simulink model "AccTarSel"  (R2018b)
settings: Solver=FixedStepDiscrete  StartTime=0.0  StopTime=inf  FixedStep=0.01  RelTol=1e-3
PostLoadFcn:
  | if any(exist('dsrtsu_mdlpostloadfcn', 'file') ~= 0), dsrtsu_mdlpostloadfcn('Execute', bdroot); end
values from neighbouring files (symbols this model uses):
  P_adtMaxBDC = 1.0    [AccTarSel.sldd]
  P_aFOCApproachIntpAcitve = -0.6    [AccTarSel.sldd]
  P_aFOCApproachIntpEnsure = -1.8    [AccTarSel.sldd]
  P_CutInEnable = 1.0    [AccTarSel.sldd]
  P_dAimMin = 4.5    [AccTarSel.sldd]
  P_dAimMinAVP = 1.5    [AccTarSel.sldd]
  P_dObjDrvOffMax = 5.0    [AccTarSel.sldd]
  P_dObjDrvOffMin = 3.0    [AccTarSel.sldd]
  P_dObjLowHystDecToStop = 4.5    [AccTarSel.sldd]
  P_dObjLowHystDecToStopAVP = 1.5    [AccTarSel.sldd]
  P_dObjUpperHystDecToStop = 5.0    [AccTarSel.sldd]
  P_dResMax = 5.0    [AccTarSel.sldd]
  P_dStandStill = 3.0    [AccTarSel.sldd]
  P_dStandStillMin = 2.0    [AccTarSel.sldd]
  P_dvarYMax4PO = 1.0    [AccTarSel.sldd]
  P_dyCutInThres = 3.6    [AccTarSel.sldd]
  P_facBDCInit = 0.7    [AccTarSel.sldd]
  P_facBDCIterCalc = 0.8    [AccTarSel.sldd]
  P_facFOCNegDiff = 0.3    [AccTarSel.sldd]
  P_facFOCPosDiff = 0.2    [AccTarSel.sldd]
  P_kapHystThres = 0.0005    [AccTarSel.sldd]
  P_PlausIntegDisable = 0.0    [AccTarSel.sldd]
  P_plausMin4PO = 0.5    [AccTarSel.sldd]
  P_probExistMin4PO = 0.8    [AccTarSel.sldd]
  P_StandObjEnable = 0.0    [AccTarSel.sldd]
  P_tAxTrackNegLower = 0.3    [AccTarSel.sldd]
  P_tAxTrackNegUpper = 0.6    [AccTarSel.sldd]
  P_tAxTrackPosLower = 1.0    [AccTarSel.sldd]
  P_tAxTrackPosUpper = 2.0    [AccTarSel.sldd]
  P_tBDCStartFilt = 0.2    [AccTarSel.sldd]
  P_tCSC = 3.5    [AccTarSel.sldd]
  P_tCurvFilt = 0.2    [AccTarSel.sldd]
  P_tCutInFilt = 0.5    [AccTarSel.sldd]
  P_tFiltAxAbsPONegFast = 0.1    [AccTarSel.sldd]
  P_tFiltAxAbsPONegSlow = 0.4    [AccTarSel.sldd]
  P_tFiltAxAbsPOPosFast = 1.2    [AccTarSel.sldd]
  P_tFiltAxAbsPOPosSlow = 2.0    [AccTarSel.sldd]
  P_tFiltAxAbsPOStand = 2.0    [AccTarSel.sldd]
  P_tFiltDAim = 0.1    [AccTarSel.sldd]
  P_tFiltDsd = 0.1    [AccTarSel.sldd]
  P_tFiltSpdLim = 3.0    [AccTarSel.sldd]
  P_tFiltVxAxPOFast = 0.15    [AccTarSel.sldd]
  P_tFiltVxAxPOSlow = 0.25    [AccTarSel.sldd]
  P_tFOCStatAccelFast = 4.0    [AccTarSel.sldd]
  P_tFOCStatAccelSlow = 3.5    [AccTarSel.sldd]
  P_tFOCStatDecelFast = 4.0    [AccTarSel.sldd]
  P_tFOCStatDecelSlow = 3.2    [AccTarSel.sldd]
  P_tMinDrvPhase = 2.0    [AccTarSel.sldd]
  P_tPredObjLeav = 1.2    [AccTarSel.sldd]
  P_tRollingFilt = 0.5    [AccTarSel.sldd]
  P_tRollingFinFilt = 1.0    [AccTarSel.sldd]
  P_tSSCNeg = 4.5    [AccTarSel.sldd]
  P_tSSCPos = 5.5    [AccTarSel.sldd]
  P_tToStop = 5.0    [AccTarSel.sldd]
  P_tToStopInBDC = 6.0    [AccTarSel.sldd]
  P_tToStopTrig = 4.0    [AccTarSel.sldd]
  P_vEgoDecToStop = 3.0    [AccTarSel.sldd]
  P_vEgoLowBDC = 4.0    [AccTarSel.sldd]
  P_vFOCNegDiff = 4.0    [AccTarSel.sldd]
  P_vFOCPosDiff = 5.0    [AccTarSel.sldd]
  P_vFOCStationaryFast = 15.0    [AccTarSel.sldd]
  P_vFOCStationarySlow = 5.0    [AccTarSel.sldd]
  P_vObjDrvOff = 0.5    [AccTarSel.sldd]
  P_vObjLowHystDecToStop = 0.5    [AccTarSel.sldd]
  P_vObjNoStop = 1.0    [AccTarSel.sldd]
  P_vObjReCalc = 1.0    [AccTarSel.sldd]
  P_vObjStop = 0.3    [AccTarSel.sldd]
  P_vObjUpperHystDecToStop = 0.8    [AccTarSel.sldd]
  P_vStandStill = 0.3    [AccTarSel.sldd]
  P_vStandStillHyst = 0.3    [AccTarSel.sldd]
  P_vyCutInThres = 0.5    [AccTarSel.sldd]
libraries: simulink x21, LPFilter x12
(part 10 of 11)

== system AccTarSel/ACC_Control/FollowObjCtrl/FollowObjValid/BrakeDistCtrl/calcCriteria/calcProfileReCalc ==
  note: should consider situation becomes urgent secnario later
  dObjToStop : Inport
  <vRef> : Inport  Port=2
  <aRef> : Inport  Port=3
  <dx> : Inport  Port=4
  vAbsObj : Inport  Port=5
  tElaps : Inport  Port=6
  BDC_StateK1 : Inport  Port=7
  ProfileK1 : Inport  Port=8
  AND : Logic  Inputs=3  AllPortsSameDT=off  OutDataTypeStr=boolean
  Abs : Abs
  Add2 : Sum  Inputs=++--
  Bus Creator : BusCreator  Inputs=5
  Bus Selector : BusSelector  OutputSignals=T30
  Constant : Constant  Value=-0.5  OutDataTypeStr=single
  Constant1 : Constant  Value=2  OutDataTypeStr=single
  Constant7 : Constant  Value=-0.3  OutDataTypeStr=single
  Constant8 : Constant  Value=2  OutDataTypeStr=single
  Divide2 : Product  Inputs=*/
  Min : MinMax  Inputs=2
  Multiply : Product
  OR : Logic  Operator=OR  Inputs=3  AllPortsSameDT=off  OutDataTypeStr=boolean
  P_dResMax : Constant  Value=P_dResMax  OutDataTypeStr=single
  P_dStandStill : Constant  Value=P_dStandStill  OutDataTypeStr=single
  P_vObjReCalc : Constant  Value=P_vObjReCalc  OutDataTypeStr=single
  Relational Operator : RelationalOperator  Operator===  OutDataTypeStr=boolean  RndMeth=Simplest
  Relational Operator1 : RelationalOperator  OutDataTypeStr=boolean  RndMeth=Simplest
  Relational Operator2 : RelationalOperator  Operator=<  OutDataTypeStr=boolean  RndMeth=Simplest
  Relational Operator4 : RelationalOperator  Operator=>  OutDataTypeStr=boolean  RndMeth=Simplest
  Relational Operator5 : RelationalOperator  Operator=>  OutDataTypeStr=boolean  RndMeth=Simplest
  Square : Math  Operator=square  SaturateOnIntegerOverflow=on
  To Workspace : ToWorkspace  VariableName=simout2  SaveFormat=Timeseries  SampleTime=-1
  ProfileReCalc : Outport
  dRes : Outport  Port=2
  wires:
  vAbsObj/1 -> Relational Operator5/1
  P_vObjReCalc/1 -> Relational Operator5/2
  P_dResMax/1 -> Relational Operator4/2
  Relational Operator5/1 -> OR/2
  P_dStandStill/1 -> Add2/4
  Add2/1 -> Relational Operator2/1, dRes/1, Bus Creator/5, Relational Operator4/1  "dRes"
  dObjToStop/1 -> Bus Creator/1, Add2/1
  Constant8/1 -> Multiply/2
  Min/1 -> Multiply/1
  <vRef>/1 -> Square/1
  Constant7/1 -> Min/2
  AND/1 -> ProfileReCalc/1
  Relational Operator4/1 -> OR/1
  Multiply/1 -> Divide2/2
  Square/1 -> Divide2/1
  <aRef>/1 -> Min/1
  <dx>/1 -> Bus Creator/2, Add2/2
  Divide2/1 -> Abs/1  "dEgoToStop"
  Abs/1 -> Add2/3
  Bus Creator/1 -> To Workspace/1
  BDC_StateK1/1 -> Relational Operator/1
  Constant1/1 -> Relational Operator/2
  ProfileK1/1 -> Bus Selector/1
  tElaps/1 -> Relational Operator1/1
  Bus Selector/1 -> Relational Operator1/2  "<T30>"
  OR/1 -> AND/1
  Relational Operator/1 -> AND/2
  Relational Operator1/1 -> AND/3, Bus Creator/4
  Constant/1 -> Relational Operator2/2
  Relational Operator2/1 -> OR/3

== system AccTarSel/ACC_Control/FollowObjCtrl/FollowObjValid/BrakeDistCtrl/calcProfile/If Action Subsystem ==
  In1 : Inport
  Action Port : ActionPort  ActionType=elseif
  Out1 : Outport
  wires:
  In1/1 -> Out1/1

== system AccTarSel/ACC_Control/FollowObjCtrl/FollowObjValid/BrakeDistCtrl/calcProfile/calc ==
  egoInfo : Inport
  objInfo : Inport  Port=2
  dObjToStop : Inport  Port=3
  aCvK1 : Inport  Port=4
  Action Port : ActionPort  ActionType=then
  Bus Creator : BusCreator  Inputs=7
  Relational Operator : RelationalOperator  OutDataTypeStr=boolean  RndMeth=Simplest
  Subsystem : Subsystem
  Switch : Switch  Criteria=u2 > Threshold
  calcInitCondition : Subsystem
  Profile : Outport
  wires:
  egoInfo/1 -> calcInitCondition/1(egoInfo)
  objInfo/1 -> calcInitCondition/2(objInfo)
  dObjToStop/1 -> calcInitCondition/3(dObjToStop)
  calcInitCondition/1(a0) -> Bus Creator/1, Switch/1, Relational Operator/1  "a0Raw"
  calcInitCondition/2(aThres) -> Switch/3, Relational Operator/2
  Relational Operator/1 -> Bus Creator/2, Switch/2  "SmoothStopCond"
  Switch/1 -> Bus Creator/3  "a0"
  calcInitCondition/3(v0) -> Bus Creator/4  "v0"
  calcInitCondition/4(v30) -> Bus Creator/5  "v30"
  calcInitCondition/5(dAimBDC) -> Bus Creator/6  "dAimBDC"
  calcInitCondition/6(d30) -> Bus Creator/7  "d30"
  Bus Creator/1 -> Subsystem/1(initCond)  "initCond"
  Subsystem/1(Profile) -> Profile/1
  aCvK1/1 -> calcInitCondition/4(aCvK1)

== system AccTarSel/ACC_Control/FollowObjCtrl/FollowObjValid/BrakeDistCtrl/calcProfile/default ==
  Action Port : ActionPort  ActionType=else
  Bus Creator : BusCreator  Inputs=8
  Constant{,1,3..7} (7 alike) : Constant  Value=0  OutDataTypeStr=single
  Constant2 : Constant  Value=0  OutDataTypeStr=boolean
  default : Outport
  wires:
  Bus Creator/1 -> default/1
  Constant1/1 -> Bus Creator/2  "aMax"
  Constant2/1 -> Bus Creator/1  "SmoothStopCond"
  Constant/1 -> Bus Creator/3  "T"
  Constant3/1 -> Bus Creator/4  "T30"
  Constant4/1 -> Bus Creator/5  "adt1"
  Constant5/1 -> Bus Creator/6  "adt2"
  Constant6/1 -> Bus Creator/7  "a0"
  Constant7/1 -> Bus Creator/8  "a0Raw"

== system AccTarSel/ACC_Control/FollowObjCtrl/FollowObjValid/FOC_MIX/Subsystem/If Action Subsystem ==
  aStat : Inport
  aApprh : Inport  Port=2
  Action Port : ActionPort  ActionType=then
  Min : MinMax  Inputs=2
  Out1 : Outport
  wires:
  aStat/1 -> Min/1
  aApprh/1 -> Min/2
  Min/1 -> Out1/1

== system AccTarSel/ACC_Control/FollowObjCtrl/FollowObjValid/FOC_MIX/Subsystem/If Action Subsystem1 ==
  aStat : Inport
  Action Port : ActionPort  ActionType=elseif
  Out1 : Outport
  wires:
  aStat/1 -> Out1/1

== system AccTarSel/ACC_Control/FollowObjCtrl/FollowObjValid/FOC_MIX/Subsystem/If Action Subsystem2 ==
  aStat : Inport
  aApprh : Inport  Port=2
  aActive : Inport  Port=3
  aEnsure : Inport  Port=4
  Action Port : ActionPort  ActionType=else
  Bus Creator : BusCreator  Inputs=2
  Bus Creator1 : BusCreator  Inputs=2
  Lookup Table Dynamic : simulink/Lookup Tables/Lookup Table Dynamic  LookUpMeth=Interpolation-Use End Values  OutDataType=fixdt('single')  OutScaling=[]  OutputDataTypeScalingMode=Specify via dialog  OutDataTypeStr=single  DoSatur=off
      settings: SourceProductName=Simulink
  Out1 : Outport
  wires:
  Bus Creator/1 -> Lookup Table Dynamic/2
  aApprh/1 -> Bus Creator1/1, Lookup Table Dynamic/1
  Bus Creator1/1 -> Lookup Table Dynamic/3
  Lookup Table Dynamic/1 -> Out1/1
  aEnsure/1 -> Bus Creator/1
  aActive/1 -> Bus Creator/2
  aStat/1 -> Bus Creator1/2

== system AccTarSel/ACC_Control/FollowObjCtrl/FollowObjValid/StationaryCtrl/calcCharactVal/If Action Subsystem ==
  dActual : Inport
  dBPNeg : Inport  Port=2
  Action Port : ActionPort  ActionType=then
  Abs : Abs
  Add : Sum  Inputs=+-
  Add1 : Sum
  Constant2 : Constant  Value=2  OutDataTypeStr=single
  Multiply : Product
  Multiply1 : Product
  Multiply2 : Product
  P_facFOCNegDiff : Constant  Value=P_facFOCNegDiff
  P_vFOCNegDiff : Constant  Value=P_vFOCNegDiff
  Sqrt : Sqrt  SaturateOnIntegerOverflow=on
  Square : Math  Operator=square  SaturateOnIntegerOverflow=on
  vUpper : Outport
  vLower : Outport  Port=2
  wires:
  dActual/1 -> Add/2
  P_facFOCNegDiff/1 -> Multiply/2
  dBPNeg/1 -> Add/1
  Sqrt/1 -> vUpper/1  "vUpper"
  Add/1 -> Multiply1/2
  Constant2/1 -> Multiply2/2
  Square/1 -> Add1/1
  Multiply2/1 -> Add1/2
  Abs/1 -> Multiply2/1
  P_vFOCNegDiff/1 -> vLower/1, Square/1, Multiply/1
  Multiply1/1 -> Abs/1
  Add1/1 -> Sqrt/1
  Multiply/1 -> Multiply1/1  "aConstNegPhase"

== system AccTarSel/ACC_Control/FollowObjCtrl/FollowObjValid/StationaryCtrl/calcCharactVal/If Action Subsystem4 ==
  dActual : Inport
  dAim : Inport  Port=2
  Action Port : ActionPort  ActionType=elseif
  Add : Sum  Inputs=+-
  Multiply : Product
  P_facFOCNegDiff : Constant  Value=P_facFOCNegDiff
  vUpper : Outport
  vLower : Outport  Port=2
  wires:
  dAim/1 -> Add/1
  dActual/1 -> Add/2
  P_facFOCNegDiff/1 -> Multiply/1
  Add/1 -> Multiply/2
  Multiply/1 -> vLower/1, vUpper/1

== system AccTarSel/ACC_Control/FollowObjCtrl/FollowObjValid/StationaryCtrl/calcCharactVal/If Action Subsystem5 ==
  dActual : Inport
  dAim : Inport  Port=2
  Action Port : ActionPort  ActionType=elseif
  Add : Sum  Inputs=+-
  Multiply : Product
  P_facFOCPosDiff : Constant  Value=P_facFOCPosDiff
  vUpper : Outport
  vLower : Outport  Port=2
  wires:
  Multiply/1 -> vUpper/1, vLower/1
  Add/1 -> Multiply/2
  P_facFOCPosDiff/1 -> Multiply/1
  dActual/1 -> Add/2
  dAim/1 -> Add/1

== system AccTarSel/ACC_Control/FollowObjCtrl/FollowObjValid/StationaryCtrl/calcCharactVal/If Action Subsystem6 ==
  dActual : Inport
  dBPPos : Inport  Port=2
  Action Port : ActionPort  ActionType=else
  Abs : Abs
  Add : Sum  Inputs=+-
  Add1 : Sum
  Constant : Constant  Value=-1  OutDataTypeStr=single
  Constant2 : Constant  Value=2  OutDataTypeStr=single
  Multiply{,1..4} (5 alike) : Product
  P_facFOCPosDiff : Constant  Value=P_facFOCPosDiff
  P_vFOCPosDiff : Constant  Value=P_vFOCPosDiff
  Sqrt : Sqrt  SaturateOnIntegerOverflow=on
  Square : Math  Operator=square  SaturateOnIntegerOverflow=on
  vUpper : Outport
  vLower : Outport  Port=2
  wires:
  Multiply/1 -> Multiply1/1  "aConstNegPhase"
  Add1/1 -> Sqrt/1
  Multiply1/1 -> Abs/1
  P_vFOCPosDiff/1 -> Multiply/1, Multiply3/1, Square/1
  Abs/1 -> Multiply2/1
  Multiply2/1 -> Add1/2
  Square/1 -> Add1/1
  Constant2/1 -> Multiply2/2
  Add/1 -> Multiply1/2
  P_facFOCPosDiff/1 -> Multiply/2
  dActual/1 -> Add/1
  dBPPos/1 -> Add/2
  Constant/1 -> Multiply3/2, Multiply4/1
  Sqrt/1 -> Multiply4/2  "vUpper"
  Multiply3/1 -> vUpper/1
  Multiply4/1 -> vLower/1

== system AccTarSel/ACC_Target_Selection/Subsystem/ValidObjCalc/CutInCalc/Subsystem/If Action Subsystem ==
  In1 : Inport
  Action Port : ActionPort  ActionType=else
  Constant : Constant  Value=0  OutDataTypeStr=single
  probCutInFiltInit : Outport
  dyCutInPredInit : Outport  Port=2
  probCutInRawInit : Outport  Port=3
  wires:
  Constant/1 -> probCutInRawInit/1, probCutInFiltInit/1
  In1/1 -> dyCutInPredInit/1

== system AccTarSel/ACC_Target_Selection/Subsystem/ValidObjCalc/CutInCalc/Subsystem/Subsystem ==
  note: MotionSts:
      | 0	Unknown
      | 1	Standstill
      | 2	Driving
      | 3	InvDriving
      | 4	Stopped
      | 5	InvStopped
  probCutInK1 : Inport
  dyToTraj : Inport  Port=2
  <vy> : Inport  Port=3
  MotionSts : Inport  Port=4
  SYS_Info_st : Inport  Port=5
  Action Port : ActionPort  ActionType=then
  Abs : Abs
  Abs1 : Abs
  Bus Selector : BusSelector  OutputSignals=dT
  Constant1 : Constant  Value=2  OutDataTypeStr=single
  Constant2 : Constant  Value=0
  If : If  IfExpression=u1 == 1
  If Action Subsystem : Subsystem  TreatAsAtomicUnit=on
  If Action Subsystem1 : Subsystem  TreatAsAtomicUnit=on
  LPFilter : LPFilter/LPFilter  SystemSampleTime=-1
      settings: SourceProductName=CustomLib
  Logical Operator : Logic  Inputs=5  AllPortsSameDT=off  OutDataTypeStr=boolean
  Merge : Merge
  Merge1 : Merge
  Multiply : Product
  P_CutInEnable : Constant  Value=P_CutInEnable
  P_dyCutInThres : Constant  Value=P_dyCutInThres
  P_tCutInFilt : Constant  Value=P_tCutInFilt
  P_vyCutInThres : Constant  Value=P_vyCutInThres
  Relational Operator : RelationalOperator  Operator=<=  OutDataTypeStr=boolean  RndMeth=Simplest
  Relational Operator1 : RelationalOperator  Operator=<  OutDataTypeStr=boolean  RndMeth=Simplest
  Relational Operator2 : RelationalOperator  Operator=>  OutDataTypeStr=boolean  RndMeth=Simplest
  Relational Operator3 : RelationalOperator  Operator===  OutDataTypeStr=boolean  RndMeth=Simplest
  probCutInFilt : Outport
  dyCutInPred : Outport  Port=2
  probCutInRaw : Outport  Port=3
  wires:
  Logical Operator/1 -> If/1
  If Action Subsystem1/1(Out1) -> Merge/2
  If Action Subsystem/2(Out2) -> Merge1/1
  P_vyCutInThres/1 -> Relational Operator2/2
  Relational Operator/1 -> Logical Operator/3
  P_CutInEnable/1 -> Logical Operator/1
  Constant2/1 -> Relational Operator1/2
  <vy>/1 -> If Action Subsystem/2(vy), Abs1/1, Multiply/2
  dyToTraj/1 -> Multiply/1, If Action Subsystem/1(dy), If Action Subsystem1/1(dy), Abs/1
  If/2 -> If Action Subsystem1/Action
  If/1 -> If Action Subsystem/Action
  Abs/1 -> Relational Operator/1
  P_dyCutInThres/1 -> Relational Operator/2
  Relational Operator2/1 -> Logical Operator/5
  Abs1/1 -> Relational Operator2/1
  If Action Subsystem1/2(Out2) -> Merge1/2
  Multiply/1 -> Relational Operator1/1
  If Action Subsystem/1(Out1) -> Merge/1
  Relational Operator1/1 -> Logical Operator/4
  Merge1/1 -> dyCutInPred/1  "dyCutInPred"
  Merge/1 -> probCutInRaw/1, LPFilter/1  "probCutIn"
  SYS_Info_st/1 -> Bus Selector/1
  Bus Selector/1 -> LPFilter/2  "<dT>"
  P_tCutInFilt/1 -> LPFilter/3
  probCutInK1/1 -> LPFilter/4
  LPFilter/1 -> probCutInFilt/1
  MotionSts/1 -> Relational Operator3/2
  Constant1/1 -> Relational Operator3/1
  Relational Operator3/1 -> Logical Operator/2

== system AccTarSel/ACC_Target_Selection/Subsystem/ValidObjCalc/TargetPlausCheck/Subsystem/CheckExistence ==
  note: logic to be expanded:
      | 1. variance threshold of dy can be interpolated according to dx
      | 2. other criteria representing existence can be added here
  In1 : Inport
  Bus Selector : BusSelector  OutputSignals=dvarY,probExist,dx
  Constant : Constant  Value=0  OutDataTypeStr=single
  Logical Operator : Logic  Inputs=3  AllPortsSameDT=off  OutDataTypeStr=boolean
  P_dvarYMax4PO : Constant  Value=P_dvarYMax4PO  OutDataTypeStr=single
  P_probExistMin4PO : Constant  Value=P_probExistMin4PO  OutDataTypeStr=single
  Relational Operator : RelationalOperator  Operator=<=  OutDataTypeStr=boolean  RndMeth=Simplest
  Relational Operator1 : RelationalOperator  OutDataTypeStr=boolean  RndMeth=Simplest
  Relational Operator2 : RelationalOperator  Operator=>  OutDataTypeStr=boolean  RndMeth=Simplest
  Out1 : Outport
  wires:
  In1/1 -> Bus Selector/1
  Bus Selector/1 -> Relational Operator/1  "<dvarY>"
  P_dvarYMax4PO/1 -> Relational Operator/2
  Bus Selector/2 -> Relational Operator1/1  "<probExist>"
  P_probExistMin4PO/1 -> Relational Operator1/2
  Relational Operator/1 -> Logical Operator/1
  Relational Operator1/1 -> Logical Operator/2
  Logical Operator/1 -> Out1/1
  Bus Selector/3 -> Relational Operator2/1  "<dx>"
  Constant/1 -> Relational Operator2/2
  Relational Operator2/1 -> Logical Operator/3

== system AccTarSel/ACC_Target_Selection/Subsystem/ValidObjCalc/TargetPlausCheck/Subsystem/CheckFOV ==
  note: logic to be expanded:
      | dx threshold can be adjusted regarding if current obj is already PO target
  In1 : Inport
  In2 : Inport  Port=2
  1-D Lookup Table : Lookup_n-D  NumberOfTableDimensions=1  LookupTableObject=''  BreakpointsForDimension1=[11.11,22.22]  BreakpointsForDimension1FirstPoint=10  BreakpointsForDimension2FirstPoint=10  BreakpointsForDimension1Spacing=12  BreakpointsForDimension2Spacing=12  IndexSearchMethod=Linear search  Table=[80,160]  ExtrapMethod=Clip  InternalRulePriority=Speed  RndMeth=Simplest  InputSameDT=on
  Bus Selector : BusSelector  OutputSignals=dx
  Bus Selector1 : BusSelector  OutputSignals=vRef
  Constant : Constant  Value=0  OutDataTypeStr=single
  Logical Operator : Logic  AllPortsSameDT=off  OutDataTypeStr=boolean
  Relational Operator : RelationalOperator  Operator=<=  OutDataTypeStr=boolean  RndMeth=Simplest
  Relational Operator1 : RelationalOperator  Operator=>  OutDataTypeStr=boolean  RndMeth=Simplest
  Out1 : Outport
  wires:
  In1/1 -> Bus Selector/1
  In2/1 -> Bus Selector1/1
  Bus Selector1/1 -> 1-D Lookup Table/1  "<vRef>"
  Bus Selector/1 -> Relational Operator1/1, Relational Operator/1  "<dx>"
  1-D Lookup Table/1 -> Relational Operator/2
  Constant/1 -> Relational Operator1/2
  Relational Operator1/1 -> Logical Operator/1
  Relational Operator/1 -> Logical Operator/2
  Logical Operator/1 -> Out1/1

== system AccTarSel/ACC_Target_Selection/Subsystem/ValidObjCalc/TargetPlausCheck/Subsystem/CheckMotSts ==
  note: MotionSts:
      | 0	Unknown
      | 1	Standstill
      | 2	Driving
      | 3	InvDriving
      | 4	Stopped
      | 5	InvStopped
  note: Type:
      | 0	Unknown
      | 1	Pedestrain
      | 2	Bi/Motor cycle
      | >=3	Vehicle
  In1 : Inport
  Bus Selector : BusSelector  OutputSignals=MotionSts,Type
  Constant : Constant  Value=2  OutDataTypeStr=single
  Constant1 : Constant  Value=4  OutDataTypeStr=single
  Constant2 : Constant  OutDataTypeStr=single
  Constant3 : Constant  Value=0  OutDataTypeStr=single
  Logical Operator1 : Logic  Operator=OR  Inputs=3  AllPortsSameDT=off  OutDataTypeStr=boolean
  Logical Operator2 : Logic  AllPortsSameDT=off  OutDataTypeStr=boolean
  P_StandObjEnable : Constant  Value=P_StandObjEnable  OutDataTypeStr=boolean
  Relational Operator : RelationalOperator  Operator===  OutDataTypeStr=boolean  RndMeth=Simplest
  Relational Operator1 : RelationalOperator  Operator===  OutDataTypeStr=boolean  RndMeth=Simplest
  Relational Operator2 : RelationalOperator  Operator===  OutDataTypeStr=boolean  RndMeth=Simplest
  Relational Operator3 : RelationalOperator  Operator=~=  OutDataTypeStr=boolean  RndMeth=Simplest
  Terminator : Terminator
  Out1 : Outport
  wires:
  In1/1 -> Bus Selector/1
  Bus Selector/1 -> Relational Operator2/1, Relational Operator1/1, Relational Operator/1  "<MotionSts>"
  Constant/1 -> Relational Operator/2
  Constant1/1 -> Relational Operator1/2
  Constant2/1 -> Relational Operator2/2
  Bus Selector/2 -> Relational Operator3/1  "<Type>"
  Constant3/1 -> Relational Operator3/2
  Relational Operator/1 -> Logical Operator1/1
  Relational Operator1/1 -> Logical Operator1/2
  Relational Operator2/1 -> Logical Operator1/3
  Logical Operator1/1 -> Logical Operator2/1
  Relational Operator3/1 -> Logical Operator2/2
  Logical Operator2/1 -> Out1/1
  P_StandObjEnable/1 -> Terminator/1

== system AccTarSel/ACC_Target_Selection/Subsystem/ValidObjCalc/TargetPlausCheck/Subsystem/CheckPlaus ==
  note: logic to be expanded:
      | plausibility threshold can be adjusted regarding if the current object is already PO target
  In1 : Inport
  P_plausMin4PO : Constant  Value=P_plausMin4PO  OutDataTypeStr=single
  Relational Operator1 : RelationalOperator  OutDataTypeStr=boolean  RndMeth=Simplest
  Out1 : Outport
  wires:
  In1/1 -> Relational Operator1/1
  P_plausMin4PO/1 -> Relational Operator1/2
  Relational Operator1/1 -> Out1/1

== system AccTarSel/ACC_Control/FollowObjCtrl/FollowObjValid/BrakeDistCtrl/calcA/If Action Subsystem/If Action Subsystem ==
  t : Inport
  a0 : Inport  Port=2
  adt1 : Inport  Port=3
  Action Port : ActionPort  ActionType=then
  Add : Sum
  Multiply : Product
  Out1 : Outport
  wires:
  t/1 -> Multiply/1
  adt1/1 -> Multiply/2
  a0/1 -> Add/1
  Multiply/1 -> Add/2
  Add/1 -> Out1/1
